simulink subsystem "Day2_Scenario_2_3"  (R2024a)
settings: Solver=VariableStepAuto  StartTime=0.0  StopTime=10.0  RelTol=1e-3
libraries: CarMaker4SL x6
settings Model: Creator=junhyung.cha  LastModifiedBy=User

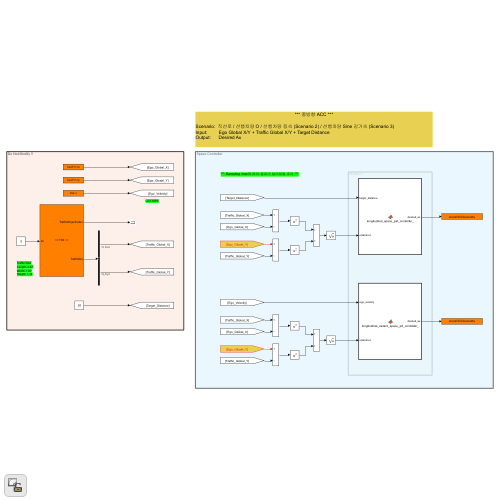
[thumbnail: Simulink's stored preview of the top-level diagram]
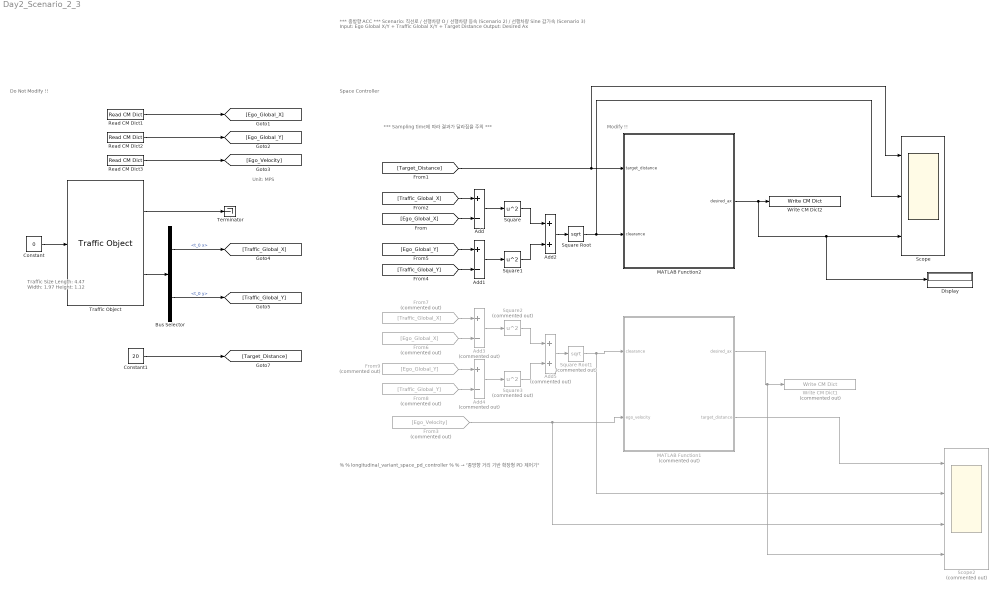
== system Day2_Scenario_2_3 ==
  note: % % longitudinal_variant_space_pd_controller
      | % % → "종방향 거리 기반 확장형 PD 제어기"
  note: *** Sampling time에 따라 결과가 달라짐을 주의 ***
  note: Space Controller
  note: Modify !!
  note: Do Not Modify !!
  note: Traffic Size
      | Length: 4.47
      | Width: 1.97
      | Height: 1.12
  note: *** 종방향 ACC ***
      |
      | Scenario: 직선로 / 선행차량 O / 선행차량 등속 (Scenario 2) / 선행차량 Sine 감가속 (Scenario 3)
      | Input: Ego Global X/Y + Traffic Global X/Y + Target Distance
      | Output: Desired Ax
  note: Unit: MPS
  Add : Sum  Inputs=+-
  Add1 : Sum  Inputs=+-
  Add2 : Sum
  Add3 : Sum  Commented=on  Inputs=+-
  Add4 : Sum  Commented=on  Inputs=+-
  Add5 : Sum  Commented=on
  Bus Selector : BusSelector  OutputSignals=t_0 x,t_0 y
  Constant : Constant  Value=0
  Constant1 : Constant  Value=20
  Display : Display
  From3 : From  Commented=on  GotoTag=Ego_Velocity
  From6 : From  Commented=on  GotoTag=Ego_Global_X
  From7 : From  Commented=on  GotoTag=Traffic_Global_X
  From8 : From  Commented=on  GotoTag=Traffic_Global_Y
  From9 : From  Commented=on  GotoTag=Ego_Global_Y
  MATLAB Function1 : MATLAB Function  Commented=on  TreatAsAtomicUnit=on
  MATLAB Function2 : MATLAB Function  TreatAsAtomicUnit=on
  Read CM Dict1 : CarMaker4SL/Read CM Dict  xname=Car.Fr1.tx  xsync=off  xstime=Inherited
  Read CM Dict2 : CarMaker4SL/Read CM Dict  xname=Car.Fr1.ty  xsync=off  xstime=Inherited
  Read CM Dict3 : CarMaker4SL/Read CM Dict  xname=Car.v  xsync=off  xstime=Inherited
  Scope : Scope  NumInputPorts=3
  Scope2 : Scope  Commented=on  NumInputPorts=4
  Square : Math  Operator=square
  Square Root : Sqrt
  Square Root1 : Sqrt  Commented=on
  Square1 : Math  Operator=square
  Square2 : Math  Commented=on  Operator=square
  Square3 : Math  Commented=on  Operator=square
  Terminator : Terminator
  Traffic Object : CarMaker4SL/Traffic Object  xname=T00  ximode=Traffic Id  xstime=Inherited
      settings: SourceProductName=CarMaker4SL
  Write CM Dict1 : CarMaker4SL/Write CM Dict  Commented=on  xname=AccelCtrl.DesiredAx  xsync=off
  Write CM Dict2 : CarMaker4SL/Write CM Dict  xname=AccelCtrl.DesiredAx  xsync=off
  wires:
  Read CM Dict2/1 -> [Ego_Global_Y]
  MATLAB Function2/1(desired_ax) -> Write CM Dict2/1, Scope/3, Display/1
  Read CM Dict1/1 -> [Ego_Global_X]
  Constant/1 -> Traffic Object/1
  Traffic Object/2 -> Bus Selector/1
  Traffic Object/1 -> Terminator/1
  Bus Selector/1 -> [Traffic_Global_X]  "<t_0 x>"
  Bus Selector/2 -> [Traffic_Global_Y]  "<t_0 y>"
  Square Root/1 -> MATLAB Function2/2(clearance), Scope/2
  Constant1/1 -> [Target_Distance]
  [Ego_Global_X] -> Add/2
  [Traffic_Global_X] -> Add/1
  [Traffic_Global_Y] -> Add1/2
  Add1/1 -> Square1/1
  Add2/1 -> Square Root/1
  Square/1 -> Add2/1
  Square1/1 -> Add2/2
  Add/1 -> Square/1
  Read CM Dict3/1 -> [Ego_Velocity]
  Add3/1 -> Square2/1
  Square3/1 -> Add5/2
  Square2/1 -> Add5/1
  Add5/1 -> Square Root1/1
  Add4/1 -> Square3/1
  From9/1 -> Add4/1
  From8/1 -> Add4/2
  From7/1 -> Add3/1
  From6/1 -> Add3/2
  MATLAB Function1/1(desired_ax) -> Write CM Dict1/1, Scope2/4
  [Target_Distance] -> MATLAB Function2/1(target_distance), Scope/1
  [Ego_Global_Y] -> Add1/1
  From3/1 -> MATLAB Function1/2(ego_velocity), Scope2/3
  Square Root1/1 -> MATLAB Function1/1(clearance), Scope2/2
  MATLAB Function1/2(target_distance) -> Scope2/1

== matlab function Day2_Scenario_2_3/MATLAB Function2 ==
  settings: updateMethod=DISCRETE  sampleTime=0.05
  data: target_distance input; desired_ax output; clearance input
% function desired_ax = longitudinal_space_pid_controller_(target_distance, clearance)
%     desired_ax = 0;
% end

function desired_ax  = longitudinal_space_pid_controller_(target_distance, clearance)
% PID 제어기: 목표 거리와 실제 거리 차이에 따른 가속도 계산

persistent prev_error integral_term initialized
dt = 0.001;  % 제어 주기 [s]

if isempty(initialized)
    prev_error = 0;
    integral_term = 0;
    initialized = true;
end

% --- PID 게인 설정 ---
Kp = 4;
Kd = 0.15;
Ki = 0.8;
% --- 오차 계산 ---
error = clearance - target_distance;
integral_term = integral_term + error * dt;
derivative = (error - prev_error) / dt;

% --- PID 제어 계산 ---
desired_ax = Kp * error + Ki * integral_term + Kd * derivative;
% desired_ax = (-1)*desired_ax 
% --- 출력 제한 (Saturation) ---
MAX_AX = 10.0;   % 일반 차량 가속 한계 (승차감 고려)
MIN_AX = -5.0;  % 일반 차량 감속 한계 (급제동 방지)

if desired_ax > MAX_AX
    desired_ax = MAX_AX;
elseif desired_ax < MIN_AX
    desired_ax = MIN_AX;
end

prev_error = error;
end

== matlab function Day2_Scenario_2_3/MATLAB Function1 ==
  settings: updateMethod=DISCRETE  sampleTime=0.05
  data: clearance input; ego_velocity input; desired_ax output; target_distance output
% function desired_ax = longitudinal_variant_space_pd_controller_(ego_velocity, clearance)
%     desired_ax = 0;
% end
%% 

% function desired_ax = longitudinal_variant_space_pd_controller_(clearance, ego_velocity)
% % PD 제어기: 거리 + 속도 기반 가속도 제어
% 
% % --- 목표 거리 ---
% target_distance = 20;  % m
% 
% % --- 상태 유지 변수 ---
% persistent prev_error
% dt = 0.001;
% 
% if isempty(prev_error)
%     prev_error = 0;
% end
% 
% % --- 오차 계산 (거리 오차 기반) ---
% error = clearance - target_distance;
% d_error = (error - prev_error) / dt;
% 
% % --- 제어기 이득 설정 ---
% Kp = 1.2;
% Kd = 0.2;
% 
% % --- 기본 PD 제어 ---
% desired_ax = Kp * error + Kd * d_error;
% 
% % --- 속도 기반 보상 (Variant) ---
% % 거리는 충분한데 Ego가 느리면 → 보조 가속
% % if error > 5 && ego_velocity < 5
% %     desired_ax = desired_ax + 1.0;
% % end
% 
% % --- 출력 제한 ---
% MAX_AX = 10.0;
% MIN_AX = -10.0;
% 
% if desired_ax > MAX_AX
%     desired_ax = MAX_AX;
% elseif desired_ax < MIN_AX
%     desired_ax = MIN_AX;
% end
% 
% prev_error = error;
% end


%% 

% function desired_ax = longitudinal_variant_space_pd_controller_(clearance, ego_velocity)
% % Constant Time Gap + PD 제어기
% % longitudinal_variant_space_pd_controller
% % → "종방향 거리 기반 확장형 PD 제어기"
% % --- 파라미터 설정 ---
% h = 1.8;  % 시간 간격 [s]
% 
% % --- 목표 거리 계산 ---
% target_distance = ego_velocity * h;
% 
% % --- 상태 변수 ---
% persistent prev_error
% dt = 0.001;
% 
% if isempty(prev_error)
%     prev_error = 0;
% end
% 
% % --- 오차 계산 ---
% error = clearance - target_distance;
% d_error = (error - prev_error) / dt;
% 
% % --- 제어기 게인 ---
% Kp = 2.0;
% Kd = 0.9;
% 
% % --- PD 제어 계산 ---
% desired_ax = Kp * error + Kd * d_error;
% 
% % --- 출력 제한 (Saturation) ---
% MAX_AX = 3.0;
% MIN_AX = -5.0;
% 
% if desired_ax > MAX_AX
%     desired_ax = MAX_AX;
% elseif desired_ax < MIN_AX
%     desired_ax = MIN_AX;
% end
% 
% % --- 상태 업데이트 ---
% prev_error = error;
% end
% 


%% 	

function [desired_ax,target_distance] = longitudinal_variant_space_pd_controller_(clearance, ego_velocity)
% Scenario 3: 선행차 Sine 감가속을 따라가는 ACC 제어기
% Constant Time Gap 모델 기반 거리 제어

% --- 파라미터 설정 ---
h = 1.8;  % 시간 간격 [sec] (headway time)
dt = 0.001;  % 샘플링 시간 [s]

% --- 목표 거리 계산 ---
target_distance = ego_velocity * h;

% --- 상태 유지 변수 ---
persistent prev_error
if isempty(prev_error)
    prev_error = 0;
end

% --- 제어 오차 계산 ---
error = clearance - target_distance;
d_error = (error - prev_error) / dt;

% --- PD 제어기 이득 설정 ---
Kp = 3;
Kd = 0.04;

% --- PD 제어 계산 ---
desired_ax = Kp * error + Kd * d_error;

% --- 출력 제한 (Saturation) ---
MAX_AX = 5.0;   % 최대 가속도 [m/s^2]
MIN_AX = -5.0;  % 최대 감속도 [m/s^2]

if desired_ax > MAX_AX
    desired_ax = MAX_AX;
elseif desired_ax < MIN_AX
    desired_ax = MIN_AX;
end

% --- 상태 업데이트 ---
prev_error = error;
end
